simulink model "ECE_431_Homework1"  (R2016a)
settings: Solver=ode1  StartTime=0.0  StopTime=20e-4  FixedStep=1e-7  RelTol=1e-3
libraries: powerlib x8
settings Model: Creator=Makenzie  LastModifiedBy=Makenzie

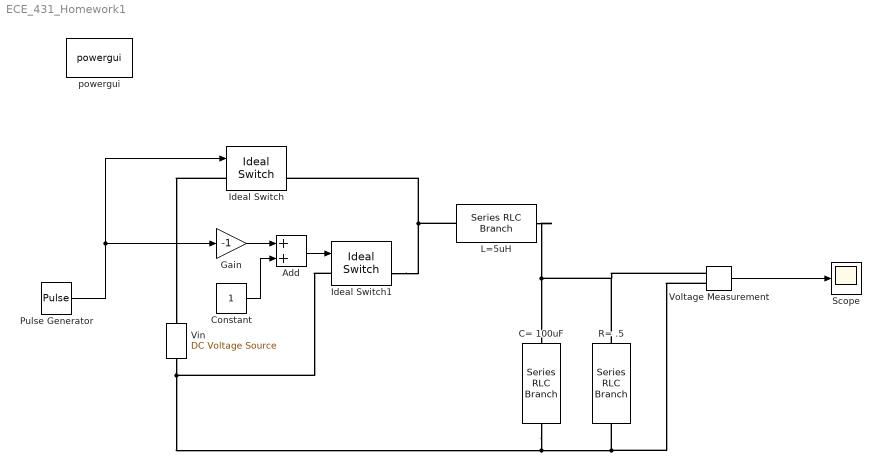
== system ECE_431_Homework1 ==
  Add : Sum
  C= 100uF : powerlib/Elements/Series RLC Branch  LConnTagsString=__new0  RConnTagsString=__new0  BranchType=RLC  Resistance=0  Inductance=0  SetiL0=off  InitialCurrent=0  Capacitance=100e-6  Setx0=off  InitialVoltage=0  Measurements=None
  Constant : Constant
  Gain : Gain  Gain=-1
  Ideal Switch : powerlib/Power Electronics/Ideal Switch  Ron=0.001  Lon=0  IC=1  Rs=1e5  Cs=inf  Measurements=on
  Ideal Switch1 : powerlib/Power Electronics/Ideal Switch  Ron=0.001  Lon=0  IC=0  Rs=1e5  Cs=inf  Measurements=on
  L=5uH : powerlib/Elements/Series RLC Branch  LConnTagsString=__new0  RConnTagsString=__new0  BranchType=RLC  Resistance=0  Inductance=5e-6  SetiL0=off  InitialCurrent=0  Capacitance=0  Setx0=off  InitialVoltage=0  Measurements=None
  Pulse Generator : DiscretePulseGenerator  PulseType=Time based  Period=1e-5  PulseWidth=75
  R= .5 : powerlib/Elements/Series RLC Branch  LConnTagsString=__new0  RConnTagsString=__new0  BranchType=RLC  Resistance=.5  Inductance=0  SetiL0=off  InitialCurrent=0  Capacitance=0  Setx0=off  InitialVoltage=0  Measurements=None
  Scope : Scope
  Vin : powerlib/Electrical Sources/DC Voltage Source  Amplitude=10  Measurements=None
  Voltage Measurement : powerlib/Measurements/Voltage Measurement  PhasorSimulation=off  OutputType=Complex  PSBequivalent=0
  powergui : powerlib/powergui  Priority=1  SimulationMode=Continuous  SolverType=Tustin/Backward Euler (TBE)  SampleTime=50e-6  frequency=60  SPID=on  DisableSnubberDevices=on  DisableRonSwitches=on  DisableVfSwitches=off  SwTol=0  DisplayEquations=off  Interpol=off  ExternalGateDelay=off  methode=off  Ts=10  FunctionMessages=off  echomessages=off  HookPort=off  EnableUseOfTLC=off  x0status=blocks  frequencyindice=0  Pbase=100e6  ErrMax=1e-4  Iterations=50  UnitsV=kV  UnitsW=MW  buscounter=0  RestoreLinks=warning  ResistiveCurrentMeasurement=off  Frange=[0:2:500]  Ylog=off  Xlog=on  ShowGrid=off  save=off  variable=ZData  structure=0  ZoomFFT=off  StartTime=0.0  cycles=1  DisplayStyle=1  fundamental=60  FreqAxis=off  MaxFrequency=1000  frequencyindicesteady=1  RmsSteady=1  display=off
  wires:
  Pulse Generator/1 -> Gain/1, Ideal Switch/1
  Add/1 -> Ideal Switch1/1
  Gain/1 -> Add/1
  Constant/1 -> Add/2
  Voltage Measurement/1 -> Scope/1
  connections:
  Ideal Switch/LConn1 -- Vin/RConn1
  Vin/LConn1 -- Ideal Switch1/LConn1 -- C= 100uF/RConn1 -- R= .5/RConn1 -- Voltage Measurement/LConn2
  L=5uH/LConn1 -- Ideal Switch1/RConn1 -- Ideal Switch/RConn1
  L=5uH/RConn1 -- R= .5/LConn1 -- Voltage Measurement/LConn1 -- C= 100uF/LConn1
